simulink model "task1_3"  (R2023a)
settings: Solver=VariableStepAuto  StartTime=0.0  StopTime=4800  RelTol=1e-3
settings Model: Creator=User  LastModifiedBy=User

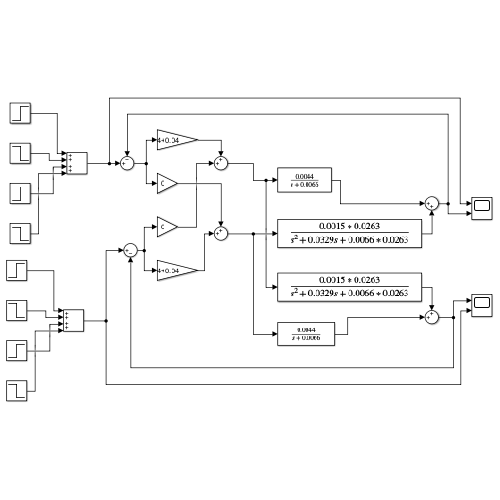
[thumbnail: Simulink's stored preview of the top-level diagram]
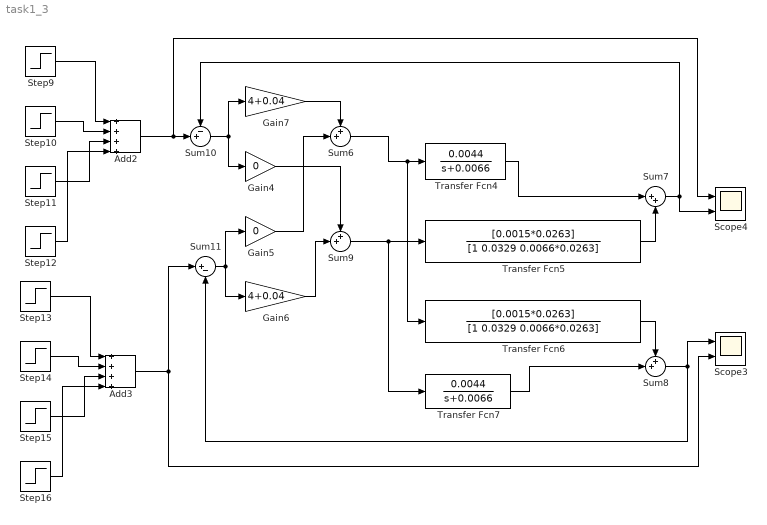
== system task1_3 ==
  Add2 : Sum  Inputs=++++
  Add3 : Sum  Inputs=++++
  Gain4 : Gain  Gain=0
  Gain5 : Gain  Gain=0
  Gain6 : Gain  Gain=4+0.04
  Gain7 : Gain  Gain=4+0.04
  Scope3 : Scope  NumInputPorts=2
  Scope4 : Scope  NumInputPorts=2
  Step10 : Step  Time=1200  After=-0.1  SampleTime=0
  Step11 : Step  Time=2400  After=0.1  SampleTime=0
  Step12 : Step  Time=3600  After=-0.1  SampleTime=0
  Step13 : Step  Time=600  After=0.1  SampleTime=0
  Step14 : Step  Time=1800  After=-0.1  SampleTime=0
  Step15 : Step  Time=3000  After=0.1  SampleTime=0
  Step16 : Step  Time=4200  After=-0.1  SampleTime=0
  Step9 : Step  Time=0  After=0.1  SampleTime=0
  Sum10 : Sum  Inputs=-+|
  Sum11 : Sum  Inputs=|+-
  Sum6 : Sum  Inputs=++|
  Sum7 : Sum  Inputs=|++
  Sum8 : Sum  Inputs=++|
  Sum9 : Sum  Inputs=++|
  Transfer Fcn4 : TransferFcn  Numerator=[0.0044]  Denominator=[1 0.0066]
  Transfer Fcn5 : TransferFcn  Numerator=[0.0015*0.0263]  Denominator=[1 0.0329 0.0066*0.0263]
  Transfer Fcn6 : TransferFcn  Numerator=[0.0015*0.0263]  Denominator=[1 0.0329 0.0066*0.0263]
  Transfer Fcn7 : TransferFcn  Numerator=[0.0044]  Denominator=[1 0.0066]
  wires:
  Add3/1 -> Sum11/1, Scope3/2
  Step12/1 -> Add2/4
  Step14/1 -> Add3/2
  Gain5/1 -> Sum6/2
  Transfer Fcn6/1 -> Sum8/1
  Gain7/1 -> Sum6/1
  Sum9/1 -> Transfer Fcn7/1, Transfer Fcn5/1
  Add2/1 -> Scope4/1, Sum10/2
  Step15/1 -> Add3/3
  Step11/1 -> Add2/3
  Step10/1 -> Add2/2
  Step9/1 -> Add2/1
  Sum7/1 -> Scope4/2, Sum10/1
  Sum6/1 -> Transfer Fcn6/1, Transfer Fcn4/1
  Sum11/1 -> Gain6/1, Gain5/1
  Sum8/1 -> Scope3/1, Sum11/2
  Transfer Fcn7/1 -> Sum8/2
  Gain4/1 -> Sum9/1
  Step13/1 -> Add3/1
  Transfer Fcn5/1 -> Sum7/2
  Transfer Fcn4/1 -> Sum7/1
  Sum10/1 -> Gain4/1, Gain7/1
  Step16/1 -> Add3/4
  Gain6/1 -> Sum9/2
